simulink library "NeuroMuscularLibrary2"  (R2019b)
settings: Solver=ode45  StartTime=0.0  StopTime=10.0  RelTol=1e-3  EnableMultiTasking=on
values from neighbouring files (symbols this model uses):
  c = 0.05    [BodyMechParams.m]
  c_jointstop = 0.3 / (pi/180)    (= 17.1887338539)    [BodyMechParams.m]
  deltaLegAngleThr = 8*pi/180    (= 0.13962634016)    [CMGParams.m]
  DeltaThRef = 2e-3    (= 0.002)    [BodyMechParams.m]
  eref = 0.04    [BodyMechParams.m]
  FmaxGLU = 1500    [BodyMechParams.m]
  footBallToAnkleDist = 0.16    [BodyMechParams.m]
  footBallToCenterDist = footLength/2    (= 0.1)    [BodyMechParams.m]
  footBallToHeelDist = footLength    (= 0.2)    [BodyMechParams.m]
  footCenterToCGDist = 0.14 - footBallToCenterDist    (= 0.04)    [BodyMechParams.m]
  footInertia = 0.005    [BodyMechParams.m]
  footLength = 0.2    [BodyMechParams.m]
  footMass = 1.25    [BodyMechParams.m]
  FT_GLU = 47.6    [BodyMechParams.m]
  g = 9.80665    [BodyMechParams.m]
  groundTheta = [atan(diff(groundZ)./diff(groundX)), 0]    [generateGround.m]
  groundZ = groundZ * stepSize/(largestStep+eps)    [generateGround.m]
  hatHipToCenterDistLen = hatLength/2    (= 0.4)    [BodyMechParams.m]
  hatInertia = 3    [BodyMechParams.m]
  hatLeftHipToCenterDistWidth = .15    (= 0.15)    [BodyMechParams.m]
  hatLength = 0.8    [BodyMechParams.m]
  hatMass = 53.5    [BodyMechParams.m]
  hatThickness = 0.2    [BodyMechParams.m]
  hatWidth = 0.4    [BodyMechParams.m]
  K = 5    [BodyMechParams.m]
  k_gn = k_gn/2    (= 39226.6)    [BodyMechParams.m]
  k_gt = k_gt/2    (= 39226.6)    [BodyMechParams.m]
  k_pressure = hatMass * g / DeltaThRef    (= 262327.8875)    [BodyMechParams.m]
  legAngleSpeedMax = 10    [CMGParams.m]
  loptGAS = 0.05    [BodyMechParams.m]
  loptGLU = 0.11    [BodyMechParams.m]
  loptHAB = 0.09    [BodyMechParams.m]
  loptHAD = 0.10    (= 0.1)    [BodyMechParams.m]
  loptHAM = 0.10    (= 0.1)    [BodyMechParams.m]
  loptHFL = 0.11    [BodyMechParams.m]
  loptSOL = 0.04    [BodyMechParams.m]
  loptTA = 0.06    [BodyMechParams.m]
  loptVAS = 0.08    [BodyMechParams.m]
  lslackGAS = 0.40    (= 0.4)    [BodyMechParams.m]
  lslackGLU = 0.13    [BodyMechParams.m]
  lslackHAB = 0.07    [BodyMechParams.m]
  lslackHAD = 0.18    [BodyMechParams.m]
  lslackHAM = 0.31    [BodyMechParams.m]
  lslackHFL = 0.10    (= 0.1)    [BodyMechParams.m]
  lslackSOL = 0.26    [BodyMechParams.m]
  lslackTA = 0.24    [BodyMechParams.m]
  lslackVAS = 0.23    [BodyMechParams.m]
  mu_slide = 0.8    [BodyMechParams.m]
  mu_stick = 0.9    [BodyMechParams.m]
  N = 1.5    [BodyMechParams.m]    (also in cmaes.m = size(x,1); mergeCompareEnergyCosts.m = {S.name})
  phiKneeUpLimit = 5*pi/180    (= 0.0872664625997)    [BodyMechParams.m]
  phimaxGASa = 20*pi/180    (= 0.349065850399)    [BodyMechParams.m]
  phimaxGASk = 40*pi/180    (= 0.698131700798)    [BodyMechParams.m]
  phimaxHAMk = 0*pi/180    (= 0)    [BodyMechParams.m]
  phimaxSOL = 20*pi/180    (= 0.349065850399)    [BodyMechParams.m]
  phimaxTA = -10*pi/180    (= -0.174532925199)    [BodyMechParams.m]
  phimaxVAS = 15*pi/180    (= 0.261799387799)    [BodyMechParams.m]
  phirefGASa = -10*pi/180    (= -0.174532925199)    [BodyMechParams.m]
  phirefGASk = 15*pi/180    (= 0.261799387799)    [BodyMechParams.m]
  phirefGLU = -30*pi/180    (= -0.523598775598)    [BodyMechParams.m]
  phirefHAB = 10*pi/180    (= 0.174532925199)    [BodyMechParams.m]
  phirefHAD = 15*pi/180    (= 0.261799387799)    [BodyMechParams.m]
  phirefHAMh = -25*pi/180    (= -0.436332312999)    [BodyMechParams.m]
  phirefHAMk = 0*pi/180    (= 0)    [BodyMechParams.m]
  phirefHFL = 0*pi/180    (= 0)    [BodyMechParams.m]
  phirefSOL = -10*pi/180    (= -0.174532925199)    [BodyMechParams.m]
  phirefTA = 20*pi/180    (= 0.349065850399)    [BodyMechParams.m]
  phirefVAS = 55*pi/180    (= 0.959931088597)    [BodyMechParams.m]
  rGASa = 0.05    [BodyMechParams.m]
  rGASk = 0.05    [BodyMechParams.m]
  rGLU = 0.10    (= 0.1)    [BodyMechParams.m]
  rHAB = 0.06    [BodyMechParams.m]
  rHAD = 0.03    [BodyMechParams.m]
  rHAMh = 0.08    [BodyMechParams.m]
  rHAMk = 0.05    [BodyMechParams.m]
  rHFL = 0.10    (= 0.1)    [BodyMechParams.m]
  rhoGASa = 0.7    [BodyMechParams.m]
  rhoGASk = 0.7    [BodyMechParams.m]
  rhoGLU = 0.5    [BodyMechParams.m]
  rhoHAB = 0.7    [BodyMechParams.m]
  rhoHAD = 1    [BodyMechParams.m]
  rhoHAMh = 0.7    [BodyMechParams.m]
  rhoHAMk = 0.7    [BodyMechParams.m]
  rhoHFL = 0.5    [BodyMechParams.m]
  rhoSOL = 0.5    [BodyMechParams.m]
  rhoTA = 0.7    [BodyMechParams.m]
  rhoVAS = 0.7    [BodyMechParams.m]
  RkneeExtendGain = 25000    [CMGParams.m]
  RkneeStopGain = 12000    [CMGParams.m]
  RlegAngleFilter = 100    [CMGParams.m]
  rSOL = 0.05    [BodyMechParams.m]
  rTA = 0.04    [BodyMechParams.m]
  rVAS = 0.06    [BodyMechParams.m]
  s = x(1:N-1,:).^2 + x(2:N,:).^2    [cmaes.m]
  shankAnkleToCenterDist = shankLength/2    (= 0.25)    [BodyMechParams.m]
  shankAnkleToKneeDist = shankLength    (= 0.5)    [BodyMechParams.m]
  shankCenterToCGDist = 0.3 - shankAnkleToCenterDist    (= 0.05)    [BodyMechParams.m]
  shankInertia = 0.05    [BodyMechParams.m]
  shankLength = 0.5    [BodyMechParams.m]
  shankMass = 3.5    [BodyMechParams.m]
  tau = 0.01    [BodyMechParams.m]
  thighCenterToCGDist = 0.3 - thighKneeToCenterDist    (= 0.05)    [BodyMechParams.m]
  thighInertia = 0.15    [BodyMechParams.m]
  thighKneeToCenterDist = thighLength/2    (= 0.25)    [BodyMechParams.m]
  thighKneeToHipDist = thighLength    (= 0.5)    [BodyMechParams.m]
  thighLength = 0.5    [BodyMechParams.m]
  thighMass = 8.5    [BodyMechParams.m]
  v_gn_max = v_gz_max    (= 0.03)    [BodyMechParams.m]
  v_gt_max = v_gz_max    (= 0.03)    [BodyMechParams.m]
  v_max_pressure = 0.5    [BodyMechParams.m]
  vLimit = 0.01    [BodyMechParams.m]
  w = 0.56    [BodyMechParams.m]    (also in MuscleEnergyTest.m = 1.039; cmaes.m = ones(size(x,1)))
  w_max_jointstop = 1 * pi/180    (= 0.0174532925199)    [BodyMechParams.m]
  X = contains(N,'compareEnergyCost') .* ~contains(N,'total') .* ~contains(N,'Total')    [mergeCompareEnergyCosts.m]
undefined symbols (not defined in the file or in its folder): abdHATRef, ankleBackDriveGain, ankleCJointstop, ankleDgain, ankleFilterPID, ankleFilterSEA, ankleGearEff, ankleGearRatio, ankleIgain, ankleInitialAngle, ankleInputMass, ankleIntCoulomb, ankleIntDamping, ankleIntStatic, ankleParallelSpringDamping, ankleParallelSpringOffset, ankleParallelSpringStiffness, anklePgain, anklePlantarLimit, ankleSEADamping, ankleSEAStiffness, ankleTendonMass, ankleWMaxJointstop, dryFrictionDamping, dryFrictionStiffness, dryFrictionVelThresh, footMassp, FourBarL1, FourBarL3, GainCHAB, GainCHAD, GainGAS, GainGLU, GainHAM, GainKneeOverExt, GainSOL, GainSOLTA, GainTA, GainVAS, hipDGain, hipDGainAbd, hipPGain, hipPGainAbd, Kglu, kneeAngleOffset, kneeBackDriveGain, kneeCJointstop, kneeDgain, kneeExtCoulomb, kneeExtDamping, kneeExtendGain, kneeExtStatic, kneeFilterPID, kneeFilterSEA, kneeFlexGain, kneeGearEff, kneeGearRatio, kneeHoldGain1, kneeHoldGain2, kneeIgain ... (+62)
libraries: sm_lib x105, nesl_utility x55, simulink x22, dspswit3 x15, $bdroot x12, simulink_extras x2
(part 4 of 6)

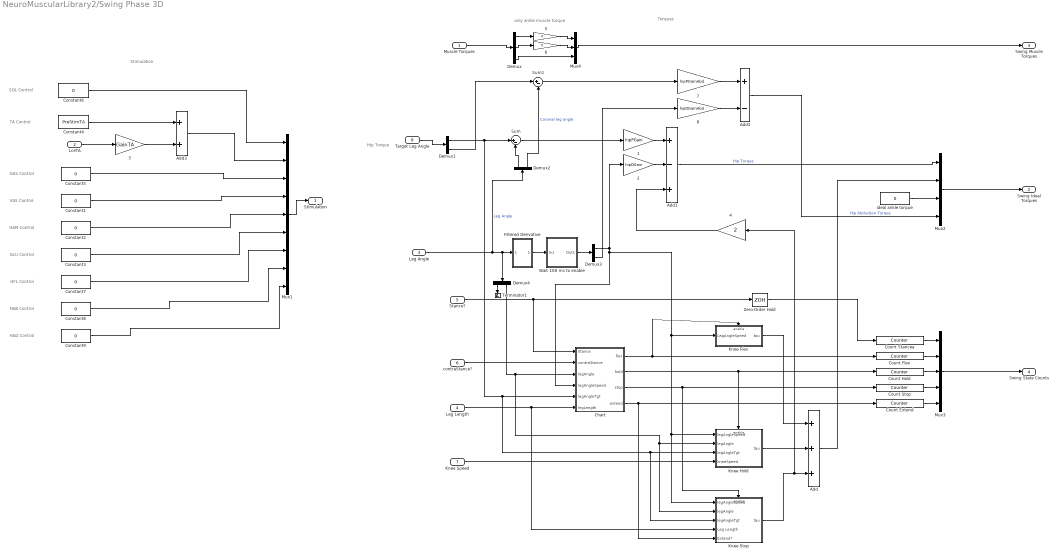
== system NeuroMuscularLibrary2/Swing Phase 3D ==
  note: only ankle muscle torque
  note: Hip Torque
  note: Torques
  note: HFL Control
  note: GLU Control
  note: HAM Control
  note: VAS Control
  note: TA Control
  note: GAS Control
  note: SOL Control
  note: Stimulation
  note: HAD Control
  note: HAB Control
  Muscle Torques : Inport
  LceTA : Inport  Port=2
  Leg Angle : Inport  Port=3
  Leg Length : Inport  Port=4
  Stance? : Inport  Port=5
  contraStance? : Inport  Port=6
  Knee Speed : Inport  Port=7
  Target Leg Angle : Inport  Port=8
  " 1" : Gain  Gain=hipPGain
  " 2" : Gain  Gain=hipDGain
  " 3" : Gain  Gain=GainTA
  " 4" : Gain  Gain=2
  " 5" : Gain  Gain=0
  " 6" : Gain  Gain=0
  " 7" : Gain  Gain=hipPGainAbd
  " 8" : Gain  Gain=hipDGainAbd
  Add : Sum  Inputs=+++
  Add1 : Sum  Inputs=+-+
  Add2 : Sum  Inputs=+-
  Add3 : Sum
  Chart : Stateflow chart  TreatAsAtomicUnit=on
  Constant{1..3,5..9} (8 alike) : Constant  Value=0
  Constant4 : Constant  Value=PreStimTA
  Count Extend : dspswit3/Counter  Direction=Up  CountEvent=Rising edge  CounterSize=16 bits  MaxCount=255  InitialCount=0  Output=Count  HitValue=32  ResetInput=off  SamplesPerFrame=1  Ts=1  CntDtype=double  HitDtype=Logical
  Count Flex : dspswit3/Counter  Direction=Up  CountEvent=Rising edge  CounterSize=16 bits  MaxCount=255  InitialCount=0  Output=Count  HitValue=32  ResetInput=off  SamplesPerFrame=1  Ts=1  CntDtype=double  HitDtype=Logical
  Count Hold : dspswit3/Counter  Direction=Up  CountEvent=Rising edge  CounterSize=16 bits  MaxCount=255  InitialCount=0  Output=Count  HitValue=32  ResetInput=off  SamplesPerFrame=1  Ts=1  CntDtype=double  HitDtype=Logical
  Count Stancea : dspswit3/Counter  Direction=Up  CountEvent=Rising edge  CounterSize=16 bits  MaxCount=255  InitialCount=0  Output=Count  HitValue=32  ResetInput=off  SamplesPerFrame=1  Ts=1  CntDtype=double  HitDtype=Logical
  Count Stop : dspswit3/Counter  Direction=Up  CountEvent=Rising edge  CounterSize=16 bits  MaxCount=255  InitialCount=0  Output=Count  HitValue=32  ResetInput=off  SamplesPerFrame=1  Ts=1  CntDtype=double  HitDtype=Logical
  Demux : Demux  Outputs=3
  Demux{1..4} (4 alike) : Demux  Outputs=2
  Filtered Derivative : Subsystem
  Knee Flex : Subsystem  TreatAsAtomicUnit=on
  Knee Hold : Subsystem  TreatAsAtomicUnit=on
  Knee Stop : Subsystem  TreatAsAtomicUnit=on
  Mux1 : Mux  Inputs=9
  Mux2 : Mux
  Mux3 : Mux  Inputs=5
  Mux4 : Mux  Inputs=3
  Sum : Sum  Inputs=|+-
  Sum1 : Sum  Inputs=|+-
  Terminator1 : Terminator
  Wait 100 ms to enable : Subsystem
  Zero-Order Hold : ZeroOrderHold  SampleTime=.01
  ideal ankle torque : Constant  Value=0
  Stimulation : Outport
  Swing Ideal Torques : Outport  Port=2
  Swing Muscle Torques : Outport  Port=3
  Swing State Counts : Outport  Port=4
  wires:
  Demux3/1 -> Chart/4(legAngleSpeed), Knee Hold/1(legAngleSpeed), Knee Stop/1(legAngleSpeed), Knee Flex/1(LegAngleSpeed), " 2"/1
  Filtered Derivative/1(Out1) -> Wait 100 ms to enable/1(In1)
  Demux1/1 -> Sum/1, Chart/5(legAngleTgt), Knee Stop/3(legAngleTgt), Knee Hold/3(legAngleTgt)
  " 2"/1 -> Add1/2
  " 1"/1 -> Add1/1
  Sum/1 -> " 1"/1
  Leg Angle/1 -> Demux4/1, Filtered Derivative/1(In1), Demux2/1  "Leg Angle"
  Mux1/1 -> Stimulation/1
  Constant7/1 -> Mux1/7
  Constant3/1 -> Mux1/6
  Constant2/1 -> Mux1/5
  Constant1/1 -> Mux1/4
  Constant5/1 -> Mux1/3
  Constant6/1 -> Mux1/1
  Add3/1 -> Mux1/2
  LceTA/1 -> " 3"/1
  " 3"/1 -> Add3/2
  Constant4/1 -> Add3/1
  Knee Speed/1 -> Knee Hold/4(kneeSpeed)
  Knee Hold/1(tau) -> Add/2
  Knee Flex/1(tau) -> Add/1
  Knee Stop/1(tau) -> " 4"/1, Add/3
  Add/1 -> Mux2/2
  " 4"/1 -> Add1/3
  Chart/1(flex) -> Knee Flex/Enable, Count Flex/1
  Chart/2(hold) -> Count Hold/1, Knee Hold/Enable
  Chart/3(stop) -> Count Stop/1, Knee Stop/Enable
  Chart/4(extend) -> Count Extend/1, Knee Stop/5(Extend?)
  Stance?/1 -> Zero-Order Hold/1, Chart/1(Stance)
  contraStance?/1 -> Chart/2(contraStance)
  Leg Length/1 -> Chart/6(legLength), Knee Stop/4(Leg Length)
  Add1/1 -> Mux2/1  "Hip Torque"
  Count Extend/1 -> Mux3/5
  Count Stop/1 -> Mux3/4
  Count Hold/1 -> Mux3/3
  Count Flex/1 -> Mux3/2
  Mux3/1 -> Swing State Counts/1
  Count Stancea/1 -> Mux3/1
  Zero-Order Hold/1 -> Count Stancea/1
  ideal ankle torque/1 -> Mux2/3
  Mux2/1 -> Swing Ideal Torques/1
  Mux4/1 -> Swing Muscle Torques/1
  Muscle Torques/1 -> Demux/1
  Demux/1 -> " 5"/1
  Demux/2 -> " 6"/1
  " 5"/1 -> Mux4/1
  " 6"/1 -> Mux4/2
  Demux/3 -> Mux4/3
  Target Leg Angle/1 -> Demux1/1
  " 8"/1 -> Add2/2
  " 7"/1 -> Add2/1
  Demux1/2 -> Sum1/1
  Sum1/1 -> " 7"/1
  Demux2/1 -> Sum/2
  Demux2/2 -> Sum1/2  "Coronal leg angle"
  Wait 100 ms to enable/1(Out1) -> Demux3/1
  Demux3/2 -> " 8"/1
  Add2/1 -> Mux2/4  "Hip Abduction Torque"
  Constant8/1 -> Mux1/8
  Constant9/1 -> Mux1/9
  Demux4/2 -> Chart/3(legAngle), Knee Stop/2(legAngle), Knee Hold/2(legAngle)
  Demux4/1 -> Terminator1/1

== system NeuroMuscularLibrary2/TA Link ==
  note: TA Attachment
  Ankle Angle [rad] : Inport
  Constant : Constant  Value=lslackTA+loptTA
  Constant2 : Constant  Value=phirefTA
  Constant3 : Constant  Value=phimaxTA
  Demux : Demux  Outputs=2
  Gain2 : Gain  Gain=rTA
  Gain4 : Gain  Gain=rhoTA
  Mux : Mux  Inputs=2
  Sum2 : Sum  Inputs=|+-
  Sum3 : Sum  Inputs=-+|
  Sum4 : Sum  Inputs=+-
  Sum5 : Sum  Inputs=|+-
  length change term : Trigonometry
  offset correction term : Trigonometry
  variable lever term : Trigonometry  Operator=cos
  lmtc [m] : Outport
  lever [m] : Outport  Port=2
  wires:
  Ankle Angle [rad]/1 -> Sum3/2
  Sum3/1 -> variable lever term/1, length change term/1
  Constant3/1 -> Sum3/1, Sum2/2
  Sum2/1 -> offset correction term/1
  Constant2/1 -> Sum2/1
  length change term/1 -> Sum4/2
  offset correction term/1 -> Sum4/1
  Sum4/1 -> Mux/1
  Constant/1 -> Sum5/1
  Sum5/1 -> lmtc [m]/1
  Gain4/1 -> Sum5/2
  variable lever term/1 -> Mux/2
  Mux/1 -> Gain2/1
  Gain2/1 -> Demux/1
  Demux/1 -> Gain4/1
  Demux/2 -> lever [m]/1

== system NeuroMuscularLibrary2/Thigh ==
  Knee to Center : sm_lib/Frames and Transforms/Rigid Transform  TranslationMethod=Cartesian  TranslationStandardOffset=0  TranslationLengthUnit=m  TranslationStandardAxis=+Z  TranslationCartesianOffset=[0 thighKneeToCenterDist 0]  TranslationROffset=0  TranslationROffsetUnits=m  TranslationZOffset=0  TranslationZOffsetUnits=m  TranslationThetaOffset=0  TranslationThetaOffsetUnits=deg  RotationMethod=AlignedAxes  RotationAngleUnits=deg  RotationStandardAxis=+Z  RotationAngle=0  RotationArbitraryAxis=[0 0 1]  FollAlignAxisA=+Z  BaseAlignAxisA=+Y  FollAlignAxisB=+X  BaseAlignAxisB=+X  RotationSequenceAxes=FollowerAxes  RotationSequence=XYX  RotationSequenceAngles=[0 0 0]  RotationSequenceAnglesUnits=deg  RotationMatrix=[1 0 0; 0 1 0; 0 0 1]
  Knee to Sensor Sheet : sm_lib/Frames and Transforms/Rigid Transform  TranslationMethod=Cartesian  TranslationStandardOffset=0  TranslationLengthUnit=m  TranslationStandardAxis=+Z  TranslationCartesianOffset=[0 thighKneeToHipDist 0]  TranslationROffset=0  TranslationROffsetUnits=m  TranslationZOffset=0  TranslationZOffsetUnits=m  TranslationThetaOffset=0  TranslationThetaOffsetUnits=deg  RotationMethod=None  RotationAngleUnits=deg  RotationStandardAxis=+Z  RotationAngle=0  RotationArbitraryAxis=[0 0 1]  FollAlignAxisA=+Z  BaseAlignAxisA=+X  FollAlignAxisB=+Y  BaseAlignAxisB=+Y  RotationSequenceAxes=FollowerAxes  RotationSequence=XYX  RotationSequenceAngles=[0 0 0]  RotationSequenceAnglesUnits=deg  RotationMatrix=[1 0 0; 0 1 0; 0 0 1]
  Thigh Center to CG : sm_lib/Frames and Transforms/Rigid Transform  TranslationMethod=Cartesian  TranslationStandardOffset=0  TranslationLengthUnit=m  TranslationStandardAxis=+Z  TranslationCartesianOffset=[0 0 thighCenterToCGDist]  TranslationROffset=0  TranslationROffsetUnits=m  TranslationZOffset=0  TranslationZOffsetUnits=m  TranslationThetaOffset=0  TranslationThetaOffsetUnits=deg  RotationMethod=None  RotationAngleUnits=deg  RotationStandardAxis=+Z  RotationAngle=0  RotationArbitraryAxis=[0 0 1]  FollAlignAxisA=+X  BaseAlignAxisA=+Y  FollAlignAxisB=+Y  BaseAlignAxisB=+Z  RotationSequenceAxes=FollowerAxes  RotationSequence=XYX  RotationSequenceAngles=[0 0 0]  RotationSequenceAnglesUnits=deg  RotationMatrix=[1 0 0; 0 1 0; 0 0 1]
  Thigh Solid : sm_lib/Body Elements/Cylindrical Solid  GraphicAmbientColor=[0.15 0.15 0.15 1.0]  BasedOnType=Density  CenterOfMass=[0 0 thighCenterToCGDist]  CenterOfMassUnits=m  GraphicDiffuseColor=[0.5 0.5 0.5]  CylinderLength=thighLength  CylinderLengthUnits=m  CylinderRadius=.075  CylinderRadiusUnits=m  Density=1000  DensityUnits=kg/(m^3)  DoExposeReferenceFrame=on  GraphicEmissiveColor=[0.0 0.0 0.0 1.0]  ExportEntireGeometry=off  SerializedFrames=<Frames/>  MarkerShape=Sphere  MarkerSize=10  GraphicType=FromGeometry  InertiaType=Custom  Mass=thighMass  MassUnits=kg  MomentsOfInertia=[thighInertia 0 0]  MomentsOfInertiaUnits=kg*m^2  GraphicOpacity=1.0  ProductsOfInertia=[0 0 0]  ProductsOfInertiaUnits=kg*m^2  GraphicShininess=75  GraphicSpecularColor=[0.5 0.5 0.5 1.0]  GraphicVisPropType=SimpleVisualProperties
  Knee : PMIOPort  Side=Left
  Sensor Sheet : PMIOPort  Port=2  Side=Right
  CG : PMIOPort  Port=3  Side=Left
  connections:
  Thigh Center to CG/RConn1 -- CG/RConn1
  Knee to Sensor Sheet/RConn1 -- Sensor Sheet/RConn1
  Thigh Center to CG/LConn1 -- Thigh Solid/RConn1 -- Knee to Center/RConn1
  Knee to Sensor Sheet/LConn1 -- Knee to Center/LConn1 -- Knee/RConn1

== system NeuroMuscularLibrary2/Torque Mixing ==
  Stance Muscle Torque : Inport
  Stance Ideal Torque : Inport  Port=2
  dxThigh : Inport  Port=3
  Stance? : Inport  Port=4
  ContraLegLeading? : Inport  Port=5
  Swing Ideal Torque : Inport  Port=6
  Swing Muscle Torque : Inport  Port=7
  Constant : Constant
  FB Gain1 : Gain  Gain=1/DeltaThRef  SaturateOnIntegerOverflow=on  OutDataTypeStr=Inherit: Same as input  ParamDataTypeStr=Inherit: Same as input
  Logical Operator : Logic  Operator=NOT  AllPortsSameDT=off  OutDataTypeStr=boolean
  Logical Operator1 : Logic  Operator=NOT  AllPortsSameDT=off  OutDataTypeStr=boolean
  Mux : Mux  Inputs=2
  Mux1 : Mux  Inputs=2
  Product{,1..3} (4 alike) : Product
  Product4 : Product  Inputs=3
  Saturation2 : Saturate  UpperLimit=1  LowerLimit=0  ZeroCross=off
  Selector : Selector  InputPortWidth=6  IndexOptions=Index vector (dialog)  Indices=[1 2 3]  OutputSizes=1
  Selector1 : Selector  InputPortWidth=6  IndexOptions=Index vector (dialog)  Indices=[4 5 6]  OutputSizes=1
  Selector3 : Selector  InputPortWidth=6  IndexOptions=Index vector (dialog)  Indices=1  OutputSizes=1
  Sum : Sum  Inputs=+|+
  Sum1 : Sum  Inputs=-+|
  Sum3 : Sum  Inputs=+++
  Hip Swing Torques : Outport  OutputWhenDisabled=reset
  Ideal Torques : Outport  Port=2  OutputWhenDisabled=reset
  Muscle Torques : Outport  Port=3  OutputWhenDisabled=reset
  wires:
  Selector3/1 -> Hip Swing Torques/1
  Sum3/1 -> Selector/1, Selector1/1
  Selector1/1 -> Muscle Torques/1
  Selector/1 -> Ideal Torques/1
  Swing Muscle Torque/1 -> Mux1/2
  Swing Ideal Torque/1 -> Mux1/1
  Stance Muscle Torque/1 -> Mux/2
  Stance Ideal Torque/1 -> Mux/1
  dxThigh/1 -> FB Gain1/1
  Mux/1 -> Product4/1, Product/1
  FB Gain1/1 -> Saturation2/1
  Saturation2/1 -> Product/2, Sum1/1
  Mux1/1 -> Product1/2, Product3/1
  Constant/1 -> Sum1/2
  Sum1/1 -> Product1/1
  Product1/1 -> Sum/2
  Product/1 -> Sum/1
  Logical Operator/1 -> Product4/3
  Stance?/1 -> Logical Operator1/1, Product4/2
  Sum/1 -> Product2/1
  Product2/1 -> Sum3/2  "Mixed Torque"
  Product4/1 -> Sum3/1  "Stance Torque Only"
  Logical Operator1/1 -> Product3/2
  Product3/1 -> Sum3/3, Selector3/1  "Swing Torque Only"
  ContraLegLeading?/1 -> Product2/2, Logical Operator/1

== system NeuroMuscularLibrary2/Upper Thigh ==
  Knee Solid : sm_lib/Body Elements/Cylindrical Solid  GraphicAmbientColor=[0.15 0.15 0.15 1.0]  BasedOnType=Density  CenterOfMass=[0 0 thighCenterToCGDist*(1-ThPos)]  CenterOfMassUnits=m  GraphicDiffuseColor=[0.5 0.5 0.5]  CylinderLength=thighLength*(1-ThPos)  CylinderLengthUnits=m  CylinderRadius=.075  CylinderRadiusUnits=m  Density=1000  DensityUnits=kg/(m^3)  DoExposeReferenceFrame=on  GraphicEmissiveColor=[0.0 0.0 0.0 1.0]  ExportEntireGeometry=off  SerializedFrames=<Frames/>  MarkerShape=Sphere  MarkerSize=10  GraphicType=FromGeometry  InertiaType=Custom  Mass=thighMass*(1-ThPos)  MassUnits=kg  MomentsOfInertia=[thighInertia*(1-ThPos)^3 0 0]  MomentsOfInertiaUnits=kg*m^2  GraphicOpacity=1.0  ProductsOfInertia=[0 0 0]  ProductsOfInertiaUnits=kg*m^2  GraphicShininess=75  GraphicSpecularColor=[0.5 0.5 0.5 1.0]  GraphicVisPropType=SimpleVisualProperties
  Knee to Center : sm_lib/Frames and Transforms/Rigid Transform  TranslationMethod=Cartesian  TranslationStandardOffset=0  TranslationLengthUnit=m  TranslationStandardAxis=+Z  TranslationCartesianOffset=[0 thighKneeToCenterDist*(1-ThPos) 0]  TranslationROffset=0  TranslationROffsetUnits=m  TranslationZOffset=0  TranslationZOffsetUnits=m  TranslationThetaOffset=0  TranslationThetaOffsetUnits=deg  RotationMethod=AlignedAxes  RotationAngleUnits=deg  RotationStandardAxis=+Z  RotationAngle=0  RotationArbitraryAxis=[0 0 1]  FollAlignAxisA=+Z  BaseAlignAxisA=+Y  FollAlignAxisB=+X  BaseAlignAxisB=+X  RotationSequenceAxes=FollowerAxes  RotationSequence=XYX  RotationSequenceAngles=[0 0 0]  RotationSequenceAnglesUnits=deg  RotationMatrix=[1 0 0; 0 1 0; 0 0 1]
  Sensor Sheet to Hip : sm_lib/Frames and Transforms/Rigid Transform  TranslationMethod=Cartesian  TranslationStandardOffset=0  TranslationLengthUnit=m  TranslationStandardAxis=+Z  TranslationCartesianOffset=[0 thighKneeToHipDist*(1-ThPos) 0]  TranslationROffset=0  TranslationROffsetUnits=m  TranslationZOffset=0  TranslationZOffsetUnits=m  TranslationThetaOffset=0  TranslationThetaOffsetUnits=deg  RotationMethod=None  RotationAngleUnits=deg  RotationStandardAxis=+Z  RotationAngle=0  RotationArbitraryAxis=[0 0 1]  FollAlignAxisA=+Z  BaseAlignAxisA=+X  FollAlignAxisB=+Y  BaseAlignAxisB=+Y  RotationSequenceAxes=FollowerAxes  RotationSequence=XYX  RotationSequenceAngles=[0 0 0]  RotationSequenceAnglesUnits=deg  RotationMatrix=[1 0 0; 0 1 0; 0 0 1]
  Thigh CG : sm_lib/Frames and Transforms/Reference Frame
  Thigh Center to CG : sm_lib/Frames and Transforms/Rigid Transform  TranslationMethod=Cartesian  TranslationStandardOffset=0  TranslationLengthUnit=m  TranslationStandardAxis=+Z  TranslationCartesianOffset=[0 0 thighCenterToCGDist*(1-ThPos)]  TranslationROffset=0  TranslationROffsetUnits=m  TranslationZOffset=0  TranslationZOffsetUnits=m  TranslationThetaOffset=0  TranslationThetaOffsetUnits=deg  RotationMethod=None  RotationAngleUnits=deg  RotationStandardAxis=+Z  RotationAngle=0  RotationArbitraryAxis=[0 0 1]  FollAlignAxisA=+X  BaseAlignAxisA=+Y  FollAlignAxisB=+Y  BaseAlignAxisB=+Z  RotationSequenceAxes=FollowerAxes  RotationSequence=XYX  RotationSequenceAngles=[0 0 0]  RotationSequenceAnglesUnits=deg  RotationMatrix=[1 0 0; 0 1 0; 0 0 1]
  Sensor Sheet : PMIOPort  Side=Left
  Hip : PMIOPort  Port=2  Side=Right
  connections:
  Sensor Sheet/RConn1 -- Knee to Center/LConn1 -- Sensor Sheet to Hip/LConn1
  Knee to Center/RConn1 -- Knee Solid/RConn1 -- Thigh Center to CG/LConn1
  Sensor Sheet to Hip/RConn1 -- Hip/RConn1
  Thigh Center to CG/RConn1 -- Thigh CG/RConn1

== system NeuroMuscularLibrary2/VAS Link ==
  note: VAS Attachment
  knee angle [rad] : Inport
  Constant : Constant  Value=lslackVAS+loptVAS
  Constant2 : Constant  Value=phirefVAS
  Constant3 : Constant  Value=phimaxVAS
  Demux : Demux  Outputs=2
  Gain2 : Gain  Gain=rVAS
  Gain4 : Gain  Gain=rhoVAS
  Mux : Mux  Inputs=2
  Sum2 : Sum  Inputs=|+-
  Sum3 : Sum  Inputs=-+|
  Sum4 : Sum  Inputs=+-
  Sum5 : Sum  Inputs=|+-
  length change term : Trigonometry
  offset correction term : Trigonometry
  variable lever term : Trigonometry  Operator=cos
  lmtu [m] : Outport
  lever [m] : Outport  Port=2
  wires:
  knee angle [rad]/1 -> Sum3/2
  Sum3/1 -> variable lever term/1, length change term/1
  Constant3/1 -> Sum3/1, Sum2/2
  Sum2/1 -> offset correction term/1
  Constant2/1 -> Sum2/1
  length change term/1 -> Sum4/2
  offset correction term/1 -> Sum4/1
  Sum4/1 -> Mux/1
  Constant/1 -> Sum5/1
  Sum5/1 -> lmtu [m]/1
  Gain4/1 -> Sum5/2
  variable lever term/1 -> Mux/2
  Mux/1 -> Gain2/1
  Gain2/1 -> Demux/1
  Demux/1 -> Gain4/1
  Demux/2 -> lever [m]/1

== system NeuroMuscularLibrary2/Full Prosthesis/Ankle  Joint ==
  Torque on Ankle : Inport
  Ankle Joint : sm_lib/Joints/Revolute Joint  JointMode=Normal  SenseConstraintForce=off  SenseConstraintForceX=off  SenseConstraintForceY=off  SenseConstraintForceZ=off  SenseConstraintTorque=off  SenseConstraintTorqueX=off  SenseConstraintTorqueY=off  SenseConstraintTorqueZ=off  SenseTotalForce=off  SenseTotalForceX=off  SenseTotalForceY=off  SenseTotalForceZ=off  SenseTotalTorque=off  SenseTotalTorqueX=off  SenseTotalTorqueY=off  SenseTotalTorqueZ=off  CompositeWrenchDir=FollowerOnBase  CompositeWrenchFrame=BaseFrame  EquilibriumPosition=0  EquilibriumPositionUnits=deg  SpringStiffness=0  SpringStiffnessUnits=N*m/rad  DampingCoefficient=0  DampingCoefficientUnits=N*m/(rad/s)  TorqueActuationMode=InputTorque  MotionActuationMode=ComputedMotion  SensePosition=on  SenseVelocity=on  SenseAcceleration=off  SenseTorqueForce=off  SenseLowerLimitTorqueForce=off  SenseUpperLimitTorqueForce=off  LowerLimitSpecify=off  LowerLimitBound=-90  LowerLimitBoundUnits=deg  LowerLimitStiffness=1e4  LowerLimitStiffnessUnits=N*m/deg  LowerLimitDamping=10  LowerLimitDampingUnits=N*m/(deg/s)  LowerLimitTransitionRegionWidth=0.1  LowerLimitTransitionRegionWidthUnits=deg  UpperLimitSpecify=off  UpperLimitBound=90  UpperLimitBoundUnits=deg  UpperLimitStiffness=1e4  UpperLimitStiffnessUnits=N*m/deg  UpperLimitDamping=10  UpperLimitDampingUnits=N*m/(deg/s)  UpperLimitTransitionRegionWidth=0.1  UpperLimitTransitionRegionWidthUnits=deg  PositionTargetSpecify=on  PositionTargetPriority=Low  PositionTargetValue=0  PositionTargetValueUnits=rad  VelocityTargetSpecify=off  VelocityTargetPriority=High  VelocityTargetValue=0  VelocityTargetValueUnits=deg/s
  Ankle Plantarflexion Limit : Subsystem  mask{phiUpLimit=anklePlantarLimit, ext=-1, c_jointstop=ankleCJointstop, w_max_jointstop=ankleWMaxJointstop}
      mask prompts: phiUpLimit "Upper Limit [rad]"; ext "Extension values are positive or negative?"; c_jointstop "Stiffness"; w_max_jointstop "Max retraction speed"
      mask help:
      | This block implements a hard joint limit that will prevent the joint from extending past the specified upper limit.
      |
      | Used for the knee and hip joints.
  PS-Simulink Converter2 : nesl_utility/PS-Simulink Converter  PhysicalDomain=network_engine_domain  SubClassName=ps_output  LeftPortType=input  RightPortType=output  PseudoPeriodic=off  Frequencies=[]  Unit=rad  AffineConversion=off
  PS-Simulink Converter3 : nesl_utility/PS-Simulink Converter  PhysicalDomain=network_engine_domain  SubClassName=ps_output  LeftPortType=input  RightPortType=output  PseudoPeriodic=off  Frequencies=[]  Unit=rad/s  AffineConversion=off
  Simulink-PS Converter : nesl_utility/Simulink-PS Converter  PhysicalDomain=network_engine_domain  SubClassName=ps_input  LeftPortType=input  RightPortType=output  PseudoPeriodic=off  Frequencies=[]  NoiseDistribution=none  NoiseParameters=[]  Unit=N*m  AffineConversion=off  FilteringAndDerivatives=zero  SimscapeFilterOrder=1  InputFilterTimeConstant=0.001  UdotUserProvided=1
  Sum : Sum  Inputs=|++
  Ankle : PMIOPort  Side=Left
  Foot : PMIOPort  Port=2  Side=Right
  Ankle Angle : Outport
  Ankle Speed : Outport  Port=2
  Actual Torque : Outport  Port=3
  Ankle Stop Torque : Outport  Port=4
  wires:
  PS-Simulink Converter3/1 -> Ankle Speed/1, Ankle Plantarflexion Limit/2(dphi [rad/s])
  Sum/1 -> Actual Torque/1, Simulink-PS Converter/1
  Torque on Ankle/1 -> Sum/1
  PS-Simulink Converter2/1 -> Ankle Angle/1, Ankle Plantarflexion Limit/1(phi [rad])
  Ankle Plantarflexion Limit/1(M_stop [Nm]) -> Sum/2, Ankle Stop Torque/1
  connections:
  Ankle Joint/LConn2 -- Simulink-PS Converter/RConn1
  Ankle Joint/RConn2 -- PS-Simulink Converter2/LConn1
  Ankle Joint/RConn3 -- PS-Simulink Converter3/LConn1
  Ankle Joint/RConn1 -- Foot/RConn1
  Ankle Joint/LConn1 -- Ankle/RConn1

== system NeuroMuscularLibrary2/Full Prosthesis/Ankle Input Joint ==
  Torque on Ankle Input : Inport
  Ankle Input Joint : sm_lib/Joints/Revolute Joint  JointMode=Normal  SenseConstraintForce=off  SenseConstraintForceX=off  SenseConstraintForceY=off  SenseConstraintForceZ=off  SenseConstraintTorque=off  SenseConstraintTorqueX=off  SenseConstraintTorqueY=off  SenseConstraintTorqueZ=off  SenseTotalForce=off  SenseTotalForceX=off  SenseTotalForceY=off  SenseTotalForceZ=off  SenseTotalTorque=off  SenseTotalTorqueX=off  SenseTotalTorqueY=off  SenseTotalTorqueZ=off  CompositeWrenchDir=FollowerOnBase  CompositeWrenchFrame=BaseFrame  EquilibriumPosition=0  EquilibriumPositionUnits=rad  SpringStiffness=0  SpringStiffnessUnits=N*m/deg  DampingCoefficient=0  DampingCoefficientUnits=N*m/(deg/s)  TorqueActuationMode=InputTorque  MotionActuationMode=ComputedMotion  SensePosition=on  SenseVelocity=on  SenseAcceleration=on  SenseTorqueForce=off  SenseLowerLimitTorqueForce=off  SenseUpperLimitTorqueForce=off  LowerLimitSpecify=off  LowerLimitBound=-90  LowerLimitBoundUnits=deg  LowerLimitStiffness=1e4  LowerLimitStiffnessUnits=N*m/deg  LowerLimitDamping=10  LowerLimitDampingUnits=N*m/(deg/s)  LowerLimitTransitionRegionWidth=0.1  LowerLimitTransitionRegionWidthUnits=deg  UpperLimitSpecify=off  UpperLimitBound=90  UpperLimitBoundUnits=deg  UpperLimitStiffness=1e4  UpperLimitStiffnessUnits=N*m/deg  UpperLimitDamping=10  UpperLimitDampingUnits=N*m/(deg/s)  UpperLimitTransitionRegionWidth=0.1  UpperLimitTransitionRegionWidthUnits=deg  PositionTargetSpecify=on  PositionTargetPriority=High  PositionTargetValue=ankleInitialAngle  PositionTargetValueUnits=rad  VelocityTargetSpecify=off  VelocityTargetPriority=High  VelocityTargetValue=0  VelocityTargetValueUnits=deg/s
  PS-Simulink Converter1 : nesl_utility/PS-Simulink Converter  PhysicalDomain=network_engine_domain  SubClassName=ps_output  LeftPortType=input  RightPortType=output  PseudoPeriodic=off  Frequencies=[]  Unit=rad/s^2  AffineConversion=off
  PS-Simulink Converter2 : nesl_utility/PS-Simulink Converter  PhysicalDomain=network_engine_domain  SubClassName=ps_output  LeftPortType=input  RightPortType=output  PseudoPeriodic=off  Frequencies=[]  Unit=rad  AffineConversion=off
  PS-Simulink Converter3 : nesl_utility/PS-Simulink Converter  PhysicalDomain=network_engine_domain  SubClassName=ps_output  LeftPortType=input  RightPortType=output  PseudoPeriodic=off  Frequencies=[]  Unit=rad/s  AffineConversion=off
  Rigid Transform : sm_lib/Frames and Transforms/Rigid Transform  TranslationMethod=None  TranslationStandardOffset=0  TranslationLengthUnit=m  TranslationStandardAxis=+Z  TranslationCartesianOffset=[0 0 0]  TranslationROffset=0  TranslationROffsetUnits=m  TranslationZOffset=0  TranslationZOffsetUnits=m  TranslationThetaOffset=0  TranslationThetaOffsetUnits=deg  RotationMethod=StandardAxis  RotationAngleUnits=deg  RotationStandardAxis=+Z  RotationAngle=180  RotationArbitraryAxis=[0 0 1]  FollAlignAxisA=+X  BaseAlignAxisA=+Y  FollAlignAxisB=+Y  BaseAlignAxisB=+Z  RotationSequenceAxes=FollowerAxes  RotationSequence=XYX  RotationSequenceAngles=[0 0 0]  RotationSequenceAnglesUnits=deg  RotationMatrix=[1 0 0; 0 1 0; 0 0 1]
  Simulink-PS Converter : nesl_utility/Simulink-PS Converter  PhysicalDomain=network_engine_domain  SubClassName=ps_input  LeftPortType=input  RightPortType=output  PseudoPeriodic=off  Frequencies=[]  NoiseDistribution=none  NoiseParameters=[]  Unit=N*m  AffineConversion=off  FilteringAndDerivatives=zero  SimscapeFilterOrder=1  InputFilterTimeConstant=0.001  UdotUserProvided=1
  Ankle Stator : PMIOPort  Side=Right
  Ankle Input : PMIOPort  Port=2  Side=Left
  Ankle Input Angle : Outport
  Ankle Input Speed : Outport  Port=2
  Ankle Input Accel : Outport  Port=3
  wires:
  PS-Simulink Converter2/1 -> Ankle Input Angle/1
  PS-Simulink Converter3/1 -> Ankle Input Speed/1
  PS-Simulink Converter1/1 -> Ankle Input Accel/1
  Torque on Ankle Input/1 -> Simulink-PS Converter/1
  connections:
  Ankle Input Joint/RConn1 -- Ankle Input/RConn1
  Ankle Input Joint/RConn3 -- PS-Simulink Converter3/LConn1
  Ankle Input Joint/RConn2 -- PS-Simulink Converter2/LConn1
  Ankle Input Joint/LConn2 -- Simulink-PS Converter/RConn1
  Ankle Input Joint/RConn4 -- PS-Simulink Converter1/LConn1
  Ankle Input Joint/LConn1 -- Rigid Transform/RConn1
  Rigid Transform/LConn1 -- Ankle Stator/RConn1

== system NeuroMuscularLibrary2/Full Prosthesis/Ankle Input Link ==
  CG : sm_lib/Frames and Transforms/Reference Frame
  Shank : sm_lib/Body Elements/File Solid  ExtGeomFileName=ankleInputLink.STL  UnitType=Custom  ExtGeomFileUnits=mm  StepReaderType=HEX  ExportEntireGeometry=off  InertiaType=Custom  Mass=ankleInputMass  MassUnits=g  CenterOfMass=ankleInputCG  CenterOfMassUnits=mm  MomentsOfInertia=ankleInputMomentOfInertia  MomentsOfInertiaUnits=g*cm^2  ProductsOfInertia=ankleInputProductOfInertia  ProductsOfInertiaUnits=g*cm^2  BasedOnType=Density  Density=1000  DensityUnits=kg/(m^3)  DoExposeReferenceFrame=on  SerializedFrames=<Frames/>  GraphicType=FromGeometry  MarkerShape=Sphere  MarkerSize=10  MarkerSizeUnits=m  GraphicVisPropType=SimpleVisualProperties  GraphicDiffuseColor=[0.5 0.5 0.5]  GraphicSpecularColor=[0.5 0.5 0.5 1.0]  GraphicAmbientColor=[0.15 0.15 0.15 1.0]  GraphicEmissiveColor=[0.0 0.0 0.0 1.0]  GraphicShininess=75  GraphicOpacity=1.0
  To CG : sm_lib/Frames and Transforms/Rigid Transform  TranslationMethod=Cartesian  TranslationStandardOffset=1.5  TranslationLengthUnit=mm  TranslationStandardAxis=-Z  TranslationCartesianOffset=ankleInputCG  TranslationROffset=0  TranslationROffsetUnits=m  TranslationZOffset=0  TranslationZOffsetUnits=m  TranslationThetaOffset=0  TranslationThetaOffsetUnits=deg  RotationMethod=None  RotationAngleUnits=deg  RotationStandardAxis=+Z  RotationAngle=0  RotationArbitraryAxis=[0 0 1]  FollAlignAxisA=+X  BaseAlignAxisA=+Y  FollAlignAxisB=+Y  BaseAlignAxisB=+Z  RotationSequenceAxes=FollowerAxes  RotationSequence=XYX  RotationSequenceAngles=[0 0 0]  RotationSequenceAnglesUnits=deg  RotationMatrix=[1 0 0; 0 1 0; 0 0 1]
  To Tendon : sm_lib/Frames and Transforms/Rigid Transform  TranslationMethod=Cartesian  TranslationStandardOffset=445.61  TranslationLengthUnit=mm  TranslationStandardAxis=-Y  TranslationCartesianOffset=[80, 0, 2]  TranslationROffset=0  TranslationROffsetUnits=m  TranslationZOffset=0  TranslationZOffsetUnits=m  TranslationThetaOffset=0  TranslationThetaOffsetUnits=deg  RotationMethod=None  RotationAngleUnits=deg  RotationStandardAxis=+Z  RotationAngle=0  RotationArbitraryAxis=[0 0 1]  FollAlignAxisA=+X  BaseAlignAxisA=+Y  FollAlignAxisB=+Y  BaseAlignAxisB=+Z  RotationSequenceAxes=FollowerAxes  RotationSequence=XYX  RotationSequenceAngles=[0 0 0]  RotationSequenceAnglesUnits=deg  RotationMatrix=[1 0 0; 0 1 0; 0 0 1]
  " Ankle Input Joint" : PMIOPort  Side=Right
  Tendon : PMIOPort  Port=2  Side=Left
  connections:
  Tendon/RConn1 -- To Tendon/RConn1
  CG/RConn1 -- To CG/RConn1
  To Tendon/LConn1 -- " Ankle Input Joint"/RConn1 -- To CG/LConn1 -- Shank/RConn1

== system NeuroMuscularLibrary2/Full Prosthesis/Ankle Motor ==
  Voltage : Inport
  Net Motor Torque : Inport  Port=2
  Load Speed : Inport  Port=3
  Ankle Motor Axis : sm_lib/Joints/Revolute Joint  JointMode=Normal  SenseConstraintForce=off  SenseConstraintForceX=off  SenseConstraintForceY=off  SenseConstraintForceZ=off  SenseConstraintTorque=off  SenseConstraintTorqueX=off  SenseConstraintTorqueY=off  SenseConstraintTorqueZ=off  SenseTotalForce=off  SenseTotalForceX=off  SenseTotalForceY=off  SenseTotalForceZ=off  SenseTotalTorque=off  SenseTotalTorqueX=off  SenseTotalTorqueY=off  SenseTotalTorqueZ=off  CompositeWrenchDir=FollowerOnBase  CompositeWrenchFrame=BaseFrame  EquilibriumPosition=0  EquilibriumPositionUnits=deg  SpringStiffness=0  SpringStiffnessUnits=N*m/deg  DampingCoefficient=0  DampingCoefficientUnits=N*m/(deg/s)  TorqueActuationMode=InputTorque  MotionActuationMode=ComputedMotion  SensePosition=on  SenseVelocity=on  SenseAcceleration=off  SenseTorqueForce=off  SenseLowerLimitTorqueForce=off  SenseUpperLimitTorqueForce=off  LowerLimitSpecify=off  LowerLimitBound=-90  LowerLimitBoundUnits=deg  LowerLimitStiffness=1e4  LowerLimitStiffnessUnits=N*m/deg  LowerLimitDamping=10  LowerLimitDampingUnits=N*m/(deg/s)  LowerLimitTransitionRegionWidth=0.1  LowerLimitTransitionRegionWidthUnits=deg  UpperLimitSpecify=off  UpperLimitBound=90  UpperLimitBoundUnits=deg  UpperLimitStiffness=1e4  UpperLimitStiffnessUnits=N*m/deg  UpperLimitDamping=10  UpperLimitDampingUnits=N*m/(deg/s)  UpperLimitTransitionRegionWidth=0.1  UpperLimitTransitionRegionWidthUnits=deg  PositionTargetSpecify=on  PositionTargetPriority=High  PositionTargetValue=-ankleInitialAngle*ankleGearRatio  PositionTargetValueUnits=rad  VelocityTargetSpecify=off  VelocityTargetPriority=High  VelocityTargetValue=0  VelocityTargetValueUnits=deg/s
  Friction : Subsystem  Commented=on  mask{Fs=ankleIntStatic, Fc=ankleIntCoulomb, sigma0=dryFrictionStiffness, sigma1=dryFrictionDamping, v_s=dryFrictionVelThresh, Fv=ankleIntDamping}
      mask prompts: Fs "Static Friction"; Fc "Colulomb Friction"; sigma0 "Dry Friction Stiffness"; sigma1 "Dry Friction Damping"; v_s "Velocity Threshold"; Fv "Viscous Friction"
  Gain : Gain  Gain=-1
  Motor Dynamics : Subsystem
  PS-Simulink Converter : nesl_utility/PS-Simulink Converter  PhysicalDomain=network_engine_domain  SubClassName=ps_output  LeftPortType=input  RightPortType=output  PseudoPeriodic=off  Frequencies=[]  Unit=rad  AffineConversion=off
  PS-Simulink Converter1 : nesl_utility/PS-Simulink Converter  PhysicalDomain=network_engine_domain  SubClassName=ps_output  LeftPortType=input  RightPortType=output  PseudoPeriodic=off  Frequencies=[]  Unit=rad/s  AffineConversion=off
  Scope : Scope  NumInputPorts=2
  Simulink-PS Converter : nesl_utility/Simulink-PS Converter  PhysicalDomain=network_engine_domain  SubClassName=ps_input  LeftPortType=input  RightPortType=output  PseudoPeriodic=off  Frequencies=[]  NoiseDistribution=none  NoiseParameters=[]  Unit=N*m  AffineConversion=off  FilteringAndDerivatives=zero  SimscapeFilterOrder=1  InputFilterTimeConstant=0.001  UdotUserProvided=1
  Sum : Sum  Inputs=+|+
  Ankle Stator : PMIOPort  Side=Right
  Ankle Rotor : PMIOPort  Port=2  Side=Left
  Motor Torque : Outport
  Motor Angle : Outport  Port=2
  Motor Speed : Outport  Port=3
  wires:
  Friction/1(Friction Force) -> Sum/2, Scope/2
  Voltage/1 -> Motor Dynamics/1(Voltage)
  PS-Simulink Converter/1 -> Motor Angle/1
  Net Motor Torque/1 -> Simulink-PS Converter/1
  PS-Simulink Converter1/1 -> Motor Dynamics/2(Speed), Motor Speed/1
  Motor Dynamics/1(Torque) -> Sum/1
  Sum/1 -> Motor Torque/1
  Load Speed/1 -> Gain/1
  Gain/1 -> Friction/1(Velocity), Scope/1
  connections:
  Ankle Motor Axis/LConn1 -- Ankle Stator/RConn1
  Ankle Motor Axis/RConn2 -- PS-Simulink Converter/LConn1
  Ankle Motor Axis/RConn3 -- PS-Simulink Converter1/LConn1
  Ankle Motor Axis/LConn2 -- Simulink-PS Converter/RConn1
  Ankle Motor Axis/RConn1 -- Ankle Rotor/RConn1

== system NeuroMuscularLibrary2/Full Prosthesis/Ankle Motor Rotor ==
  CG : sm_lib/Frames and Transforms/Reference Frame
  Knee Rotor1 : sm_lib/Body Elements/File Solid  ExtGeomFileName=motorRotor.STL  UnitType=Custom  ExtGeomFileUnits=mm  StepReaderType=HEX  ExportEntireGeometry=off  InertiaType=Custom  Mass=motorRotorMass  MassUnits=g  CenterOfMass=motorRotorCG  CenterOfMassUnits=mm  MomentsOfInertia=motorRotorMomentOfInertia  MomentsOfInertiaUnits=g*cm^2  ProductsOfInertia=motorRotorProductOfInertia  ProductsOfInertiaUnits=g*cm^2  BasedOnType=Density  Density=1000  DensityUnits=kg/(m^3)  DoExposeReferenceFrame=on  SerializedFrames=<Frames/>  GraphicType=FromGeometry  MarkerShape=Sphere  MarkerSize=10  MarkerSizeUnits=m  GraphicVisPropType=SimpleVisualProperties  GraphicDiffuseColor=[0.5 0.5 0.5]  GraphicSpecularColor=[0.5 0.5 0.5 1.0]  GraphicAmbientColor=[0.15 0.15 0.15 1.0]  GraphicEmissiveColor=[0.0 0.0 0.0 1.0]  GraphicShininess=75  GraphicOpacity=1.0
  Rigid Transform : sm_lib/Frames and Transforms/Rigid Transform  TranslationMethod=StandardAxis  TranslationStandardOffset=4.5  TranslationLengthUnit=mm  TranslationStandardAxis=+Z  TranslationCartesianOffset=[0 0 0]  TranslationROffset=0  TranslationROffsetUnits=m  TranslationZOffset=0  TranslationZOffsetUnits=m  TranslationThetaOffset=0  TranslationThetaOffsetUnits=deg  RotationMethod=None  RotationAngleUnits=deg  RotationStandardAxis=+Z  RotationAngle=0  RotationArbitraryAxis=[0 0 1]  FollAlignAxisA=+X  BaseAlignAxisA=+Y  FollAlignAxisB=+Y  BaseAlignAxisB=+Z  RotationSequenceAxes=FollowerAxes  RotationSequence=XYX  RotationSequenceAngles=[0 0 0]  RotationSequenceAnglesUnits=deg  RotationMatrix=[1 0 0; 0 1 0; 0 0 1]
  ToCG : sm_lib/Frames and Transforms/Rigid Transform  TranslationMethod=Cartesian  TranslationStandardOffset=0  TranslationLengthUnit=mm  TranslationStandardAxis=+Z  TranslationCartesianOffset=motorRotorCG  TranslationROffset=0  TranslationROffsetUnits=m  TranslationZOffset=0  TranslationZOffsetUnits=m  TranslationThetaOffset=0  TranslationThetaOffsetUnits=deg  RotationMethod=None  RotationAngleUnits=deg  RotationStandardAxis=+Z  RotationAngle=0  RotationArbitraryAxis=[0 0 1]  FollAlignAxisA=+X  BaseAlignAxisA=+Y  FollAlignAxisB=+Y  BaseAlignAxisB=+Z  RotationSequenceAxes=FollowerAxes  RotationSequence=XYX  RotationSequenceAngles=[0 0 0]  RotationSequenceAnglesUnits=deg  RotationMatrix=[1 0 0; 0 1 0; 0 0 1]
  Conn1 : PMIOPort  Side=Right
  connections:
  CG/RConn1 -- ToCG/RConn1
  ToCG/LConn1 -- Knee Rotor1/RConn1 -- Rigid Transform/RConn1
  Conn1/RConn1 -- Rigid Transform/LConn1

== system NeuroMuscularLibrary2/Full Prosthesis/Ankle Parallel Spring ==
  Ankle Angle : Inport
  Ankle Speed : Inport  Port=2
  Add : Sum
  Bias : Bias  Bias=-ankleParallelSpringOffset
  Parallel Spring Stiffness : Gain  Gain=-ankleParallelSpringStiffness
  Parallel Spring Damping : Gain  Gain=-ankleParallelSpringDamping
  Saturation1 : Saturate  UpperLimit=0  LowerLimit=-inf  ZeroCross=off
  Saturation2 : Saturate  UpperLimit=0  LowerLimit=-inf  ZeroCross=off
  Parallel Spring Torque : Outport
  wires:
  Add/1 -> Parallel Spring Torque/1
  Ankle Speed/1 -> Parallel Spring Damping/1
  Parallel Spring Stiffness/1 -> Saturation2/1
  Parallel Spring Damping/1 -> Saturation1/1
  Bias/1 -> Parallel Spring Stiffness/1
  Ankle Angle/1 -> Bias/1
  Saturation1/1 -> Add/2
  Saturation2/1 -> Add/1

== system NeuroMuscularLibrary2/Full Prosthesis/Ankle SEA Control ==
  Motor Speed : Inport
  Load Acceleration : Inport  Port=2
  Measured Torque : Inport  Port=3
  Desired Ankle Torque : Inport  Port=4
  Parallel Spring Torque : Inport  Port=5
  Ankle Input Angle : Inport  Port=6
  Tendon Angle : Inport  Port=7
  Ankle Angle : Inport  Port=8
  4 bar ratio : Subsystem
  Divide : Product  Inputs=*/
  Feed Forward : Subsystem
  PID Controller : simulink/Continuous/PID Controller  Controller=PD  Form=Parallel  TimeDomain=Continuous-time  SampleTime=-1  IntegratorMethod=Forward Euler  FilterMethod=Forward Euler  ControllerParametersSource=internal  P=anklePgain  I=ankleIgain  D=ankleDgain  UseFilter=on  N=ankleFilterPID  TunerSelectOption=Transfer Function Based (PID Tuner App)  InitialConditionSource=internal  InitialConditionForIntegrator=0  InitialConditionForFilter=0  DifferentiatorICPrevScaledInput=0  ExternalReset=none  TrackingMode=off  Kt=1  LimitOutput=off  UpperSaturationLimit=inf  LowerSaturationLimit=-inf  LinearizeAsGain=on  AntiWindupMode=none  Kb=1  POutMin=[]  POutMax=[]  IOutMin=[]  IOutMax=[]  DOutMin=[]  DOutMax=[]  NOutMin=[]  NOutMax=[]  SumOutMin=[]  SumOutMax=[]  SaturationOutMin=[]  SaturationOutMax=[]  PParamMin=[]  PParamMax=[]  IParamMin=[]  IParamMax=[]  DParamMin=[]  DParamMax=[]  NParamMin=[]  NParamMax=[]  KbParamMin=[]  KbParamMax=[]  KtParamMin=[]  KtParamMax=[]  KbOutMin=[]  KbOutMax=[]  KtOutMin=[]  KtOutMax=[]  IntegratorOutMin=[]  IntegratorOutMax=[]  FilterOutMin=[]  FilterOutMax=[]  SumI1OutMin=[]  SumI1OutMax=[]  SumI2OutMin=[]  SumI2OutMax=[]  SumI3OutMin=[]  SumI3OutMax=[]  SumI4OutMin=[]  SumI4OutMax=[]  SumDOutMin=[]  SumDOutMax=[]  DifferentiatorOutMin=[]  DifferentiatorOutMax=[]  FilterDiffOutCoefMin=[]  FilterDiffOutCoefMax=[]  ReciprocalOutMin=[]  ReciprocalOutMax=[]  SumDenOutMin=[]  SumDenOutMax=[]  SumNumOutMin=[]  SumNumOutMax=[]  DivideOutMin=[]  DivideOutMax=[]  IntegratorContinuousStateAttributes=''  IntegratorStateMustResolveToSignalObject=off  IntegratorRTWStateStorageClass=Auto  FilterContinuousStateAttributes=''  FilterStateMustResolveToSignalObject=off  FilterRTWStateStorageClass=Auto  ParallelPVariant=InternalParameters  IdealPVariant=Disabled  IVariant=Disabled  DVariant=InternalParameters  IntegratorVariant=Disabled  SatVariant=Disabled  AWVariant=Disabled  PCopyVariant=Disabled  TRVariant=Disabled  FdbkBlocksVariant=Forward  IdealPFdbkVariant=Disabled  SatFdbkVariant=Disabled  DerivativeFilterVariant=ContFilter  NVariant=InternalParameters  NCopyVariant=Disabled  FilterICVariant=InternalICsFilter  IntegratorICVariant=Disabled  ExternalResetVariant=Disabled  TRSumVariant=Passthrough  SumFdbkVariant=Disabled  SumVariant=Sum_PD
  Saturation1 : Saturate  UpperLimit=motorMaxVoltage  LowerLimit=-motorMaxVoltage  ZeroCross=off
  Sum : Sum  Inputs=|+-
  Sum1 : Sum  Inputs=+-|
  Sum2 : Sum  Inputs=|+-
  Motor Voltage : Outport
  Desired Actuator Torque : Outport  Port=2
  wires:
  Divide/1 -> Sum/1, Feed Forward/3(Desired Actuator Torque), Desired Actuator Torque/1  "Desired Actuator"
  Sum2/1 -> Divide/1
  Saturation1/1 -> Motor Voltage/1
  Sum1/1 -> Saturation1/1
  Load Acceleration/1 -> Feed Forward/2(Load Acceleration)
  Ankle Input Angle/1 -> 4 bar ratio/1(Ankle Input Angle)
  Tendon Angle/1 -> 4 bar ratio/2(Tendon Angle)
  Ankle Angle/1 -> 4 bar ratio/3(Ankle Angle)
  Measured Torque/1 -> Sum/2
  Sum/1 -> PID Controller/1
  4 bar ratio/1(ratio) -> Divide/2
  Motor Speed/1 -> Feed Forward/1(Motor Speed)
  Feed Forward/1(Computed Motor Voltage) -> Sum1/1
  Desired Ankle Torque/1 -> Sum2/1
  Parallel Spring Torque/1 -> Sum2/2
  PID Controller/1 -> Sum1/2
